simulink model "testboardinternalADC"  (R2018b)
settings: Solver=FixedStepDiscrete  StartTime=0.0  StopTime=Inf  RelTol=1e-3  EnableMultiTasking=on
undefined symbols (not defined in the file or in its folder): Down, GPTRIP1SEL, GPTRIP2SEL, TZ1, TZ2, Up
libraries: c2837xDlib x19, c2802xlib x3, c2000lib x1, simulink x1
settings Model: ExtModeTrigDuration=8  Creator=ThinkPad  LastModifiedBy=ThinkPad
settings OptimizationCC: DefaultUnderspecifiedDataType=single  EnhancedBackFolding=on  PassReuseOutputArgsAs=Individual arguments  MaxStackSize=512  OptimizeBlockOrder=speed  DifferentSizesBufferReuse=on  OptimizationCustomize=off
settings DebuggingCC: ParameterTunabilityLossMsg=error
settings HardwareCC: ProdBitPerChar=16  ProdBitPerInt=16  ProdBitPerPointer=32  ProdBitPerSizeT=32  ProdBitPerPtrDiffT=32  ProdLargestAtomicInteger=Integer  ProdLargestAtomicFloat=None  ProdWordSize=16  ProdLongLongMode=on  ProdHWDeviceType=Texas Instruments->C2000  TargetBitPerChar=16  TargetBitPerInt=16  TargetLargestAtomicInteger=Integer  TargetLongLongMode=on  TargetIntDivRoundTo=Zero  TargetEndianess=LittleEndian  TargetWordSize=16  TargetHWDeviceType=Texas Instruments->C2000
settings SFSimCC: MATLABDynamicMemAlloc=off
settings RTWCC: SystemTargetFile=ert.tlc  HardwareBoard=TI Delfino F2837xD  GenCodeOnly=on  TemplateMakefile=ert_default_tmf  GenerateReport=on  CustomInclude=C:\Users\ThinkPad\Desktop\MBDCODE\  CustomSource=F2837xD_Emif.c  Toolchain=Texas Instruments Code Composer Studio (C2000)  IncludeHyperlinkInReport=on  LaunchReport=on  GenerateTraceInfo=on  GenerateTraceReport=on  GenerateTraceReportSl=on  GenerateTraceReportSf=on  GenerateTraceReportEml=on
settings RTWCC: CustomSourceCode=|
  | //
  | // Globals
  | //
  | Uint16  ErrCount = 0;
  | Uint32  TEST_STATUS;
  | int i;
  | 
  | //
  | // Function Prototypes
  | //
  | extern void setup_emif1_pinmux_async_16bit(Uint16);
  | extern void Emif1Initialize(void);
  | //
  | // mem_read_write - This function performs simple read/write word accesses
  | //                  to memory.
  | //
  | char
  | mem_read_write(Uint32 start_addr, Uint32 mem_size)
  | {
  |     unsigned long mem_rds;
  |     unsigned long mem_wds;
  |     long *XMEM_ps;
  |     unsigned int i;
  | 
  |     //
  |     //Write data
  |     //
  |     XMEM_ps = (long *)start_addr;
  | 
  |     //
  |     //Fill memory
  |     //
  |     mem_wds = 0x01234567;
  |     for (i=0; i < mem_size; i++)
  |     {
  |         *XMEM_ps++ = mem_wds;
  |         mem_wds += 0x11111111;
  |     }
  | 
  |     //
  |     //Verify memory
  |     //
  |     mem_wds = 0x01234567;
  |     XMEM_ps = (long *)start_addr;
  |     for (i=0; i < mem_size; i++)
  |     {
  |         mem_rds = *XMEM_ps;
  |         if( mem_rds != mem_wds)
  |         {
  |             return(1);
  |         }
  |         XMEM_ps++;
  |         mem_wds += 0x11111111;
  |     }
  |     return(0);
  | }
  | 
  | //
  | //  mem_data_walk - This function performs a walking 0 & 1 on data lines for
  | //                  SRAM RD & WR
  | //
  | char
  | mem_data_walk(Uint32 start_addr, Uint32 mem_size)
  | {
  |     unsigned long sram_rd;
  |     unsigned long sram_wd;
  |     unsigned long i;
  |     int k;
  |     int m;
  |     unsigned long  *XM_p;
  |     unsigned long  *XMEM_p;
  | 
  |     XM_p = (unsigned long *)start_addr;
  | 
  |     for (i=0; i < mem_size; i=i+64)
  |     {
  |         for (m=0; m < 2; m++)
  |         {
  |             //
  |             //Write loop
  |             //
  |             XMEM_p = XM_p;
  |             sram_wd = 0x01;
  |             for (k=0; k < 32; k++)
  |             {
  |                 if(m==0)
  |                 {
  |                     *XMEM_p++ =  sram_wd;
  |                 }
  |                 else
  |                 {
  |                     *XMEM_p++ = ~sram_wd;
  |                 }
  |                 sram_wd   = sram_wd<<1;
  |             }
  | 
  |             //
  |             //Read loop
  |             //
  |             XMEM_p = XM_p;
  |             sram_wd = 0x01;
  |             for (k=0; k < 32; k++)
  |             {
  |                 sram_rd = *XMEM_p;
  |                 if(m==1)
  |                 {
  |                     sram_rd = ~sram_rd;
  |                 }
  |                 if(sram_rd != sram_wd)
  |                 {
  |                     return(1);
  |                 }
  |                 XMEM_p++;
  |                 sram_wd=sram_wd<<1;
  |             }
  |         }
  |         XM_p = XMEM_p;
  |     }
  |     return(0);
  | }
  | 
  | //
  | // mem_addr_walk - This function performs a toggle on each address bit.
  | //
  | char
  | mem_addr_walk(Uint32 start_addr, Uint32 addr_size)
  | {
  |     unsigned long sram_rd;
  |     unsigned long sram_wd;
  |     unsigned int k;
  |     unsigned long xshift;
  |     unsigned long  *XM_p;
  |     unsigned long  *XMEM_p;
  | 
  |     XM_p = (unsigned long *)start_addr;
  | 
  |     //
  |     //Write loop
  |     //
  |     xshift = 0x00000001;
  |     sram_wd = 0x00;
  |     for (k=0; k < addr_size; k++)
  |     {
  |         XMEM_p = (unsigned long *)(start_addr + xshift);
  |         *XMEM_p = sram_wd++;
  |         xshift = xshift<<1;
  |     }
  | 
  |     //
  |     //Read loop
  |     //
  |     XMEM_p = XM_p;
  |     xshift = 0x00000001;
  |     sram_wd = 0x00;
  |     for (k=0; k < addr_size; k++)
  |     {
  |         XMEM_p = (unsigned long *)(start_addr + xshift);
  |         sram_rd = *XMEM_p;
  |        if(sram_rd != sram_wd)
  |        {
  |            return(1);
  |        }
  | 
  |        xshift = xshift<<1;
  |        sram_wd++;
  |     }
  |     return(0);
  | }
  | 
  | //
  | // mem_data_size - This function performs different data type
  | //                (HALFWORD/WORD) access.
  | //
  | char
  | mem_data_size(Uint32 start_addr, Uint32 size_to_check)
  | {
  |     unsigned short mem_rds;
  |     unsigned long  mem_rdl;
  |     unsigned short mem_wds;
  |     unsigned long  mem_wdl;
  |     int i;
  | 
  |     short *XMEM_ps;
  |     long  *XMEM_pl;
  | 
  |     //
  |     //Write data short
  |     //
  |     XMEM_ps = (short *)start_addr;
  |     mem_wds = 0x0605;
  | 
  |     for (i=0; i < 2; i++)
  |     {
  |         *XMEM_ps++ = mem_wds;
  |         mem_wds += 0x0202;
  |     }
  | 
  |     //
  |     //Write data long
  |     //
  |     XMEM_pl = (long *)XMEM_ps;
  |     mem_wdl = 0x0C0B0A09;
  |     for (i=0; i < 2; i++)
  |     {
  |         *XMEM_pl++ = mem_wdl;
  |         mem_wdl += 0x04040404;
  |     }
  | 
  |     //
  |     //Read data short
  |     //
  |     XMEM_ps = (short *)start_addr;
  |     mem_wds = 0x0605;
  |     for (i=0; i < 6; i++)
  |     {
  |         mem_rds = *XMEM_ps;
  |         if( mem_rds != mem_wds)
  |         {
  |             return(1);
  |         }
  |         XMEM_ps++;
  |         mem_wds += 0x0202;
  |     }
  | 
  |     //
  |     //Read data long
  |     //
  |     XMEM_pl = (long *)start_addr;
  |     mem_wdl = 0x08070605;
  |     for (i=0; i < 3; i++)
  |     {
  |         mem_rdl = *XMEM_pl;
  |         if(mem_rdl != mem_wdl)
  |         {
  |             return(1);
  |         }
  |         XMEM_pl++;
  |         mem_wdl += 0x04040404;
  |     }
  |     return(0);
  | }
settings RTWCC: CustomHeaderCode=|
  | #include "F28x_Project.h"
  | 
  | #define TEST_PASS            0xABCDABCD
  | #define TEST_FAIL            0xDEADDEAD
  | #define ASRAM_CS3_START_ADDR 0x100000
  | #define ASRAM_CS3_SIZE       0x8000
  | //#define EMIF1                0
  | //#define EMIF2                1
  | #define MEM_D_WIDTH          1            // 16Bit Memory Interface
  | #define TURN_AROUND_TIME     0            // Turn Around time of 2 Emif Clock
  | #define RD_SETUP_TIME        0            // Read Setup time of 1 Emif Clock
  | #define RD_STROBE_TIME       3            // Read Strobe time of 4 Emif Clock
  | #define RD_HOLD_TIME         0            // Read Hold time of 1 Emif Clock
  | #define WR_SETUP_TIME        0            // Write Hold time of 1 Emif Clock
  | #define WR_STROBE_TIME       0            // Write Setup time of 1 Emif Clock
  | #define WR_HOLD_TIME         0            // Write Hold time of 1 Emif Clock
  | #define EXTEND_WAIT          0            // Disable Extended Wait
  | #define STROBE_SEL           0            // Disable Strobe Mode.
  | #define WAIT_POLAR_INV       0
  | #define WAIT_COUNT           0
settings RTWCC: CustomInitializer=|
  | char ErrCount_local;
  |   TEST_STATUS = TEST_FAIL;
  | 
  |   Emif1Initialize();
  |   EALLOW;
  |   CpuSysRegs.PCLKCR1.bit.EMIF1 = 1;
  |   CpuSysRegs.PCLKCR1.bit.EMIF2 = 0;
  |   EDIS;
  |   EALLOW;
  |   ClkCfgRegs.PERCLKDIVSEL.bit.EMIF1CLKDIV = 0x1;
  |   EDIS;
  | 
  |  EALLOW;
  |   ClkCfgRegs.PERCLKDIVSEL.bit.EMIF1CLKDIV = 0x0;
  |   EDIS;
  | 
  |   EALLOW;
  | //
  | // Grab EMIF1 For CPU1
  | //
  |   Emif1ConfigRegs.EMIF1MSEL.all = 0x93A5CE71;
  |   if(Emif1ConfigRegs.EMIF1MSEL.all != 0x1)
  |   {
  |       ErrCount++;
  |   }
  | 
  | //
  | //Disable Access Protection (CPU_FETCH/CPU_WR/DMA_WR)
  | //
  |   Emif1ConfigRegs.EMIF1ACCPROT0.all = 0x0;
  |   if(Emif1ConfigRegs.EMIF1ACCPROT0.all != 0x0)
  |   {
  |       ErrCount++;
  |   }
  | 
  | //
  | // Commit the configuration related to protection. Till this bit remains set
  | // content of EMIF1ACCPROT0 register can't be changed.
  | //
  |   Emif1ConfigRegs.EMIF1COMMIT.all = 0x1;
  |   if(Emif1ConfigRegs.EMIF1COMMIT.all != 0x1)
  |   {
  |      ErrCount++;
  |   }
  | 
  | //
  | // Lock the configuration so that EMIF1COMMIT register can't be
  | // changed any more.
  | //
  |   Emif1ConfigRegs.EMIF1LOCK.all = 0x1;
  |   if(Emif1ConfigRegs.EMIF1LOCK.all != 1)
  |   {
  |       ErrCount++;
  |   }
  | 
  |   EDIS;
  | 
  | 
  | 
  |   EALLOW;
  |   Emif1Regs.RCSR.bit.MODULE_ID = 0x000F;
  |   Emif1Regs.RCSR.bit.FR =1;
  |   EDIS;
  |   EALLOW;
  |   Emif1Regs.ASYNC_WCCR.bit.WP0 = 1;
  |   Emif1Regs.ASYNC_WCCR.bit.MAX_EXT_WAIT = 80;
  |   EDIS;
  |   EALLOW;
  |   Emif1Regs.INT_MSK_SET.bit.AT_MASK_SET = 1;
  |   EDIS;
  | 
  | 
  |     Uint16 i;
  |     for (i=28; i<=37;i++)
  |     {
  |         GPIO_SetupPinMux(i,0,2);
  |     }
  |     for (i=69; i<=83;i++)
  |     {
  |         GPIO_SetupPinMux(i,0,2);
  |     }
  | 
  |     //setup async mode and enable pull-ups for Data pins
  |     for (i=69; i<=83;i++)
  |     {
  |         GPIO_SetupPinOptions(i,0,0x31); // GPIO_ASYNC||GPIO_PULLUP
  |     }
  | 
  | //Configure GPIO pins for EMIF1
  | //
  | //Configure the access timing for CS2 space
  | Emif1Regs.ASYNC_CS3_CR.all =  (EMIF_ASYNC_ASIZE_16    | // 16Bit Memory Interface
  |                              EMIF_ASYNC_TA_4    | // Turn Around time of 2 Emif Clock
  |                              EMIF_ASYNC_RHOLD_4   | // Read Hold time of 1 Emif Clock
  |                              EMIF_ASYNC_RSTROBE_13   | // Read Strobe time of 4 Emif Clock
  |                              EMIF_ASYNC_RSETUP_2  | // Read Setup time of 1 Emif Clock
  |                              EMIF_ASYNC_WHOLD_2   | // Write Hold time of 1 Emif Clock
  |                              EMIF_ASYNC_WSTROBE_7   | // Write Strobe time of 1 Emif Clock
  |                              EMIF_ASYNC_WSETUP_3 | // Write Setup time of 1 Emif Clock
  |                              EMIF_ASYNC_EW_ENABLE  | // Extended Wait Disable.
  |                              EMIF_ASYNC_SS_DISABLE    // Strobe Select Mode Disable.
  |                             );
  | 
  |   ErrCount_local = mem_read_write(ASRAM_CS3_START_ADDR, ASRAM_CS3_SIZE);
  |   ErrCount = ErrCount + ErrCount_local;
  | 
  | //
  | //Address walk checks (Tested for Memory with address width of 16bit)
  | //
  |   ErrCount_local = mem_addr_walk(ASRAM_CS3_START_ADDR, 16);
  |   ErrCount = ErrCount + ErrCount_local;
  | 
  | //
  | //Data walk checks
  | //
  |   ErrCount_local = mem_data_walk(ASRAM_CS3_START_ADDR, ASRAM_CS3_SIZE);
  |   ErrCount = ErrCount + ErrCount_local;
  | 
  | //
  | //Data size checks
  | //
  |   ErrCount_local = mem_data_size(ASRAM_CS3_START_ADDR, 4);
  |   ErrCount = ErrCount + ErrCount_local;
  | 
  |   if (ErrCount == 0x0)
  |   {
  |       TEST_STATUS = TEST_PASS;
  |   }
settings CodeAppCC: ForceParamTrailComments=on  IgnoreCustomStorageClasses=off  OperatorAnnotations=on  SimulinkDataObjDesc=on  SFDataObjDesc=on  InsertBlockDesc=on
settings ERTTargetCC: CodeReplacementLibrary=TI C28x

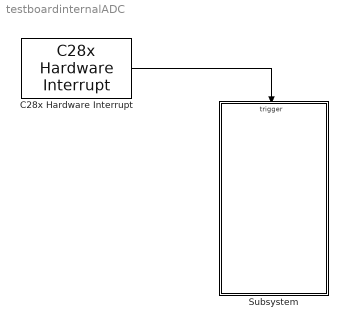
== system testboardinternalADC ==
  C28x Hardware Interrupt : c2000lib/Scheduling/C28x Hardware Interrupt  irqnumbers=[3 3]  pienumbers=[1 2]  irqpriorities=[30 26]  irqpreempts=[0 0]  showinput=off  dspchiptype=C280X
      settings: SourceProductName=Embedded Coder Support Package for Texas Instruments C2000 Processors  SourceProductBaseCode=TIC2000
  Subsystem : Subsystem
  wires:
  C28x Hardware Interrupt/1 -> Subsystem/Trigger

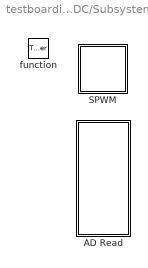
== system testboardinternalADC/Subsystem ==
  function : TriggerPort  TriggerType=function-call  VariantControl=(inherit)  SampleTime=1e-5
  AD Read : Subsystem
  SPWM : Subsystem

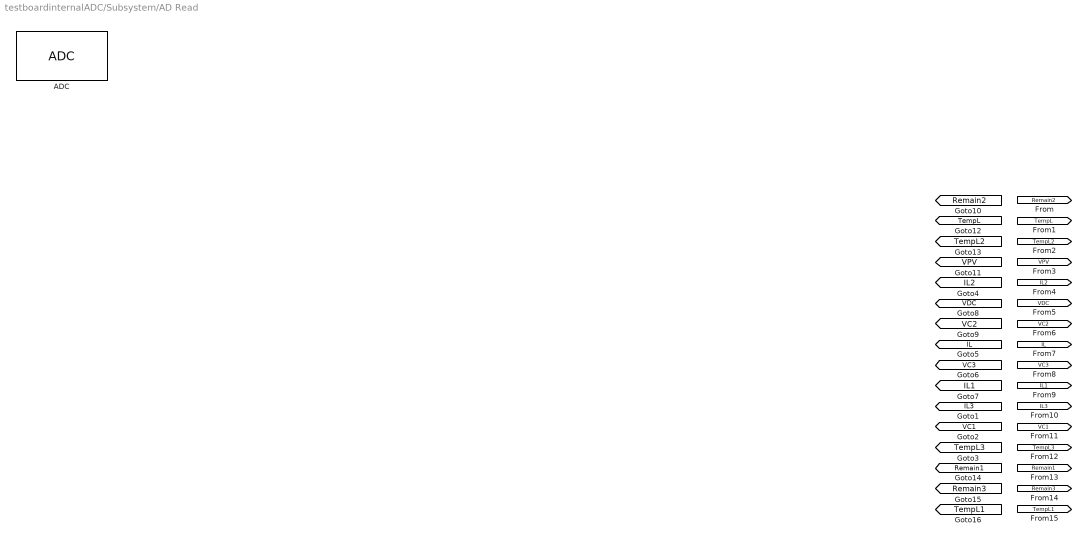
== system testboardinternalADC/Subsystem/AD Read ==
  ADC : c2802xlib/ADC  ADCModule=A  samplingMode=Single sample mode  ADCResolution=12-bit (Single-ended input)  useSOC1=SOC0  useSOC2=SOC0_SOC1  SOCAcquisitionWindow=15  SOCTriggerSource=Software  SOCInterruptTrigger=ADCINT1  Ts=0.001  dType=uint16  postInterrupt=off  interruptSel=ADCINT1  ADCINTContinuous=on  endma=off  chdma=1  blkParamProc=C2000_Type4  conv1=ADCINA0  conv2=ADCINA0 and ADCINB0  conv1_Type4=ADCIN0  conv2_Type4=ADCIN0 and ADCIN1
      settings: SourceProductName=Embedded Coder Support Package for Texas Instruments C2000 Processors
  tag scope: IL1=global, IL2=global, IL3=global, IL=global, Remain1=global, Remain2=global, Remain3=global, TempL1=global, TempL2=global, TempL3=global, TempL=global, VC1=global, VC2=global, VC3=global, VDC=global, VPV=global
  wires:
  ? -> [TempL1]
  ? -> [Remain3]
  ? -> [Remain1]
  ? -> [TempL3]
  ? -> [VC1]
  ? -> [IL1]
  ? -> [VC3]
  ? -> [VC2]
  ? -> [VDC]
  ? -> [TempL2]
  ? -> [IL]
  ? -> [TempL]
  ? -> [VPV]
  ? -> [Remain2]
  ? -> [IL2]
  ? -> [IL3]

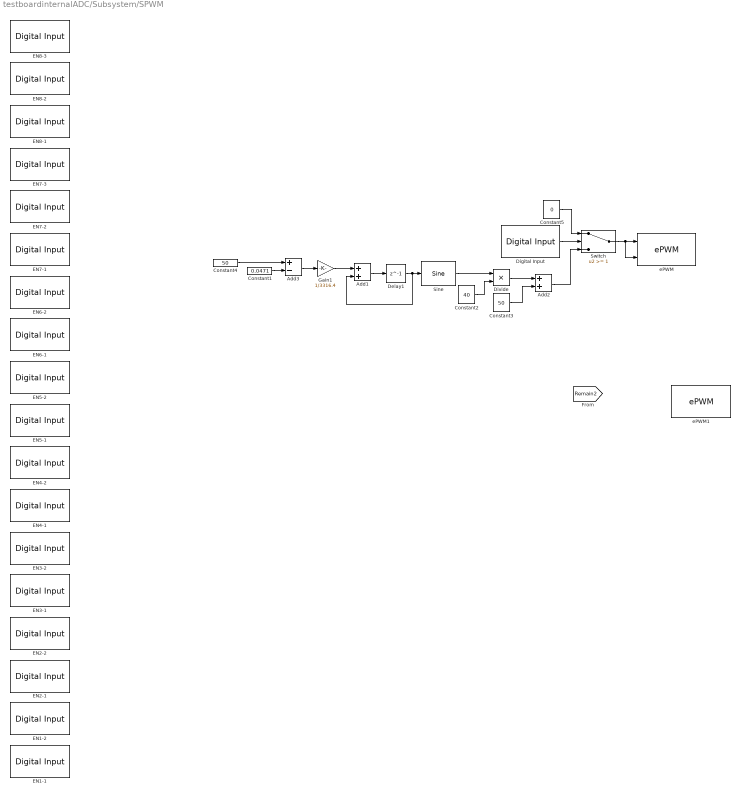
== system testboardinternalADC/Subsystem/SPWM ==
  Add1 : Sum
  Add2 : Sum
  Add3 : Sum  Inputs=+-
  Constant1 : Constant  Value=0.0471  VectorParams1D=off
  Constant2 : Constant  Value=40  VectorParams1D=off
  Constant3 : Constant  Value=50  VectorParams1D=off
  Constant4 : Constant  Value=50  VectorParams1D=off
  Constant5 : Constant  Value=0  VectorParams1D=off
  Delay1 : Delay  DelayLength=1
  Digital Input : c2837xDlib/Digital Input  GPIO_Number=GPIO96~GPIO103  GPIO_Bit0=off  GPIO_Bit1=off  GPIO_Bit2=off  GPIO_Bit3=on  GPIO_Bit4=off  GPIO_Bit5=off  GPIO_Bit6=off  GPIO_Bit7=off  sampleTime=-1  dataType=auto  GPIO_Bit0_Qualification=Sync to SYSCLKOUT  GPIO_Bit1_Qualification=Sync to SYSCLKOUT  GPIO_Bit2_Qualification=Sync to SYSCLKOUT  GPIO_Bit3_Qualification=Sync to SYSCLKOUT  GPIO_Bit4_Qualification=Sync to SYSCLKOUT  GPIO_Bit5_Qualification=Sync to SYSCLKOUT  GPIO_Bit6_Qualification=Sync to SYSCLKOUT  GPIO_Bit7_Qualification=Sync to SYSCLKOUT  Qualification_Period=-1
      settings: SourceProductName=Embedded Coder Support Package for Texas Instruments C2000 Processors  SourceProductBaseCode=TIC2000
  Divide : Product  Inputs=**
  EN1-1 : c2837xDlib/Digital Input  GPIO_Number=GPIO88~GPIO95  GPIO_Bit0=off  GPIO_Bit1=off  GPIO_Bit2=on  GPIO_Bit3=off  GPIO_Bit4=off  GPIO_Bit5=off  GPIO_Bit6=off  GPIO_Bit7=off  sampleTime=0.1  dataType=auto  GPIO_Bit0_Qualification=Sync to SYSCLKOUT  GPIO_Bit1_Qualification=Sync to SYSCLKOUT  GPIO_Bit2_Qualification=Sync to SYSCLKOUT  GPIO_Bit3_Qualification=Sync to SYSCLKOUT  GPIO_Bit4_Qualification=Sync to SYSCLKOUT  GPIO_Bit5_Qualification=Sync to SYSCLKOUT  GPIO_Bit6_Qualification=Sync to SYSCLKOUT  GPIO_Bit7_Qualification=Sync to SYSCLKOUT  Qualification_Period=-1
      settings: SourceProductName=Embedded Coder Support Package for Texas Instruments C2000 Processors  SourceProductBaseCode=TIC2000
  EN1-2 : c2837xDlib/Digital Input  GPIO_Number=GPIO88~GPIO95  GPIO_Bit0=off  GPIO_Bit1=on  GPIO_Bit2=off  GPIO_Bit3=off  GPIO_Bit4=off  GPIO_Bit5=off  GPIO_Bit6=off  GPIO_Bit7=off  sampleTime=0.1  dataType=auto  GPIO_Bit0_Qualification=Sync to SYSCLKOUT  GPIO_Bit1_Qualification=Sync to SYSCLKOUT  GPIO_Bit2_Qualification=Sync to SYSCLKOUT  GPIO_Bit3_Qualification=Sync to SYSCLKOUT  GPIO_Bit4_Qualification=Sync to SYSCLKOUT  GPIO_Bit5_Qualification=Sync to SYSCLKOUT  GPIO_Bit6_Qualification=Sync to SYSCLKOUT  GPIO_Bit7_Qualification=Sync to SYSCLKOUT  Qualification_Period=-1
      settings: SourceProductName=Embedded Coder Support Package for Texas Instruments C2000 Processors  SourceProductBaseCode=TIC2000
  EN2-1 : c2837xDlib/Digital Input  GPIO_Number=GPIO88~GPIO95  GPIO_Bit0=on  GPIO_Bit1=off  GPIO_Bit2=off  GPIO_Bit3=off  GPIO_Bit4=off  GPIO_Bit5=off  GPIO_Bit6=off  GPIO_Bit7=off  sampleTime=0.1  dataType=auto  GPIO_Bit0_Qualification=Sync to SYSCLKOUT  GPIO_Bit1_Qualification=Sync to SYSCLKOUT  GPIO_Bit2_Qualification=Sync to SYSCLKOUT  GPIO_Bit3_Qualification=Sync to SYSCLKOUT  GPIO_Bit4_Qualification=Sync to SYSCLKOUT  GPIO_Bit5_Qualification=Sync to SYSCLKOUT  GPIO_Bit6_Qualification=Sync to SYSCLKOUT  GPIO_Bit7_Qualification=Sync to SYSCLKOUT  Qualification_Period=-1
      settings: SourceProductName=Embedded Coder Support Package for Texas Instruments C2000 Processors  SourceProductBaseCode=TIC2000
  EN2-2 : c2837xDlib/Digital Input  GPIO_Number=GPIO80~GPIO87  GPIO_Bit0=off  GPIO_Bit1=off  GPIO_Bit2=off  GPIO_Bit3=off  GPIO_Bit4=off  GPIO_Bit5=off  GPIO_Bit6=off  GPIO_Bit7=on  sampleTime=0.1  dataType=auto  GPIO_Bit0_Qualification=Sync to SYSCLKOUT  GPIO_Bit1_Qualification=Sync to SYSCLKOUT  GPIO_Bit2_Qualification=Sync to SYSCLKOUT  GPIO_Bit3_Qualification=Sync to SYSCLKOUT  GPIO_Bit4_Qualification=Sync to SYSCLKOUT  GPIO_Bit5_Qualification=Sync to SYSCLKOUT  GPIO_Bit6_Qualification=Sync to SYSCLKOUT  GPIO_Bit7_Qualification=Sync to SYSCLKOUT  Qualification_Period=-1
      settings: SourceProductName=Embedded Coder Support Package for Texas Instruments C2000 Processors  SourceProductBaseCode=TIC2000
  EN3-1 : c2837xDlib/Digital Input  GPIO_Number=GPIO80~GPIO87  GPIO_Bit0=off  GPIO_Bit1=off  GPIO_Bit2=off  GPIO_Bit3=off  GPIO_Bit4=off  GPIO_Bit5=off  GPIO_Bit6=on  GPIO_Bit7=off  sampleTime=0.1  dataType=auto  GPIO_Bit0_Qualification=Sync to SYSCLKOUT  GPIO_Bit1_Qualification=Sync to SYSCLKOUT  GPIO_Bit2_Qualification=Sync to SYSCLKOUT  GPIO_Bit3_Qualification=Sync to SYSCLKOUT  GPIO_Bit4_Qualification=Sync to SYSCLKOUT  GPIO_Bit5_Qualification=Sync to SYSCLKOUT  GPIO_Bit6_Qualification=Sync to SYSCLKOUT  GPIO_Bit7_Qualification=Sync to SYSCLKOUT  Qualification_Period=-1
      settings: SourceProductName=Embedded Coder Support Package for Texas Instruments C2000 Processors  SourceProductBaseCode=TIC2000
  EN3-2 : c2837xDlib/Digital Input  GPIO_Number=GPIO48~GPIO55  GPIO_Bit0=off  GPIO_Bit1=off  GPIO_Bit2=off  GPIO_Bit3=off  GPIO_Bit4=on  GPIO_Bit5=off  GPIO_Bit6=off  GPIO_Bit7=off  sampleTime=0.1  dataType=auto  GPIO_Bit0_Qualification=Sync to SYSCLKOUT  GPIO_Bit1_Qualification=Sync to SYSCLKOUT  GPIO_Bit2_Qualification=Sync to SYSCLKOUT  GPIO_Bit3_Qualification=Sync to SYSCLKOUT  GPIO_Bit4_Qualification=Sync to SYSCLKOUT  GPIO_Bit5_Qualification=Sync to SYSCLKOUT  GPIO_Bit6_Qualification=Sync to SYSCLKOUT  GPIO_Bit7_Qualification=Sync to SYSCLKOUT  Qualification_Period=-1
      settings: SourceProductName=Embedded Coder Support Package for Texas Instruments C2000 Processors  SourceProductBaseCode=TIC2000
  EN4-1 : c2837xDlib/Digital Input  GPIO_Number=GPIO48~GPIO55  GPIO_Bit0=off  GPIO_Bit1=off  GPIO_Bit2=off  GPIO_Bit3=on  GPIO_Bit4=off  GPIO_Bit5=off  GPIO_Bit6=off  GPIO_Bit7=off  sampleTime=0.1  dataType=auto  GPIO_Bit0_Qualification=Sync to SYSCLKOUT  GPIO_Bit1_Qualification=Sync to SYSCLKOUT  GPIO_Bit2_Qualification=Sync to SYSCLKOUT  GPIO_Bit3_Qualification=Sync to SYSCLKOUT  GPIO_Bit4_Qualification=Sync to SYSCLKOUT  GPIO_Bit5_Qualification=Sync to SYSCLKOUT  GPIO_Bit6_Qualification=Sync to SYSCLKOUT  GPIO_Bit7_Qualification=Sync to SYSCLKOUT  Qualification_Period=-1
      settings: SourceProductName=Embedded Coder Support Package for Texas Instruments C2000 Processors  SourceProductBaseCode=TIC2000
  EN4-2 : c2837xDlib/Digital Input  GPIO_Number=GPIO48~GPIO55  GPIO_Bit0=off  GPIO_Bit1=off  GPIO_Bit2=on  GPIO_Bit3=off  GPIO_Bit4=off  GPIO_Bit5=off  GPIO_Bit6=off  GPIO_Bit7=off  sampleTime=0.1  dataType=auto  GPIO_Bit0_Qualification=Sync to SYSCLKOUT  GPIO_Bit1_Qualification=Sync to SYSCLKOUT  GPIO_Bit2_Qualification=Sync to SYSCLKOUT  GPIO_Bit3_Qualification=Sync to SYSCLKOUT  GPIO_Bit4_Qualification=Sync to SYSCLKOUT  GPIO_Bit5_Qualification=Sync to SYSCLKOUT  GPIO_Bit6_Qualification=Sync to SYSCLKOUT  GPIO_Bit7_Qualification=Sync to SYSCLKOUT  Qualification_Period=-1
      settings: SourceProductName=Embedded Coder Support Package for Texas Instruments C2000 Processors  SourceProductBaseCode=TIC2000
  EN5-1 : c2837xDlib/Digital Input  GPIO_Number=GPIO48~GPIO55  GPIO_Bit0=off  GPIO_Bit1=on  GPIO_Bit2=off  GPIO_Bit3=off  GPIO_Bit4=off  GPIO_Bit5=off  GPIO_Bit6=off  GPIO_Bit7=off  sampleTime=0.1  dataType=auto  GPIO_Bit0_Qualification=Sync to SYSCLKOUT  GPIO_Bit1_Qualification=Sync to SYSCLKOUT  GPIO_Bit2_Qualification=Sync to SYSCLKOUT  GPIO_Bit3_Qualification=Sync to SYSCLKOUT  GPIO_Bit4_Qualification=Sync to SYSCLKOUT  GPIO_Bit5_Qualification=Sync to SYSCLKOUT  GPIO_Bit6_Qualification=Sync to SYSCLKOUT  GPIO_Bit7_Qualification=Sync to SYSCLKOUT  Qualification_Period=-1
      settings: SourceProductName=Embedded Coder Support Package for Texas Instruments C2000 Processors  SourceProductBaseCode=TIC2000
  EN5-2 : c2837xDlib/Digital Input  GPIO_Number=GPIO48~GPIO55  GPIO_Bit0=on  GPIO_Bit1=off  GPIO_Bit2=off  GPIO_Bit3=off  GPIO_Bit4=off  GPIO_Bit5=off  GPIO_Bit6=off  GPIO_Bit7=off  sampleTime=0.1  dataType=auto  GPIO_Bit0_Qualification=Sync to SYSCLKOUT  GPIO_Bit1_Qualification=Sync to SYSCLKOUT  GPIO_Bit2_Qualification=Sync to SYSCLKOUT  GPIO_Bit3_Qualification=Sync to SYSCLKOUT  GPIO_Bit4_Qualification=Sync to SYSCLKOUT  GPIO_Bit5_Qualification=Sync to SYSCLKOUT  GPIO_Bit6_Qualification=Sync to SYSCLKOUT  GPIO_Bit7_Qualification=Sync to SYSCLKOUT  Qualification_Period=-1
      settings: SourceProductName=Embedded Coder Support Package for Texas Instruments C2000 Processors  SourceProductBaseCode=TIC2000
  EN6-1 : c2837xDlib/Digital Input  GPIO_Number=GPIO40~GPIO47  GPIO_Bit0=off  GPIO_Bit1=off  GPIO_Bit2=off  GPIO_Bit3=off  GPIO_Bit4=off  GPIO_Bit5=off  GPIO_Bit6=off  GPIO_Bit7=on  sampleTime=0.1  dataType=auto  GPIO_Bit0_Qualification=Sync to SYSCLKOUT  GPIO_Bit1_Qualification=Sync to SYSCLKOUT  GPIO_Bit2_Qualification=Sync to SYSCLKOUT  GPIO_Bit3_Qualification=Sync to SYSCLKOUT  GPIO_Bit4_Qualification=Sync to SYSCLKOUT  GPIO_Bit5_Qualification=Sync to SYSCLKOUT  GPIO_Bit6_Qualification=Sync to SYSCLKOUT  GPIO_Bit7_Qualification=Sync to SYSCLKOUT  Qualification_Period=-1
      settings: SourceProductName=Embedded Coder Support Package for Texas Instruments C2000 Processors  SourceProductBaseCode=TIC2000
  EN6-2 : c2837xDlib/Digital Input  GPIO_Number=GPIO40~GPIO47  GPIO_Bit0=off  GPIO_Bit1=off  GPIO_Bit2=off  GPIO_Bit3=off  GPIO_Bit4=off  GPIO_Bit5=off  GPIO_Bit6=on  GPIO_Bit7=off  sampleTime=0.1  dataType=auto  GPIO_Bit0_Qualification=Sync to SYSCLKOUT  GPIO_Bit1_Qualification=Sync to SYSCLKOUT  GPIO_Bit2_Qualification=Sync to SYSCLKOUT  GPIO_Bit3_Qualification=Sync to SYSCLKOUT  GPIO_Bit4_Qualification=Sync to SYSCLKOUT  GPIO_Bit5_Qualification=Sync to SYSCLKOUT  GPIO_Bit6_Qualification=Sync to SYSCLKOUT  GPIO_Bit7_Qualification=Sync to SYSCLKOUT  Qualification_Period=-1
      settings: SourceProductName=Embedded Coder Support Package for Texas Instruments C2000 Processors  SourceProductBaseCode=TIC2000
  EN7-1 : c2837xDlib/Digital Input  GPIO_Number=GPIO40~GPIO47  GPIO_Bit0=off  GPIO_Bit1=off  GPIO_Bit2=off  GPIO_Bit3=off  GPIO_Bit4=off  GPIO_Bit5=on  GPIO_Bit6=off  GPIO_Bit7=off  sampleTime=0.1  dataType=auto  GPIO_Bit0_Qualification=Sync to SYSCLKOUT  GPIO_Bit1_Qualification=Sync to SYSCLKOUT  GPIO_Bit2_Qualification=Sync to SYSCLKOUT  GPIO_Bit3_Qualification=Sync to SYSCLKOUT  GPIO_Bit4_Qualification=Sync to SYSCLKOUT  GPIO_Bit5_Qualification=Sync to SYSCLKOUT  GPIO_Bit6_Qualification=Sync to SYSCLKOUT  GPIO_Bit7_Qualification=Sync to SYSCLKOUT  Qualification_Period=-1
      settings: SourceProductName=Embedded Coder Support Package for Texas Instruments C2000 Processors  SourceProductBaseCode=TIC2000
  EN7-2 : c2837xDlib/Digital Input  GPIO_Number=GPIO40~GPIO47  GPIO_Bit0=off  GPIO_Bit1=off  GPIO_Bit2=off  GPIO_Bit3=off  GPIO_Bit4=on  GPIO_Bit5=off  GPIO_Bit6=off  GPIO_Bit7=off  sampleTime=0.1  dataType=auto  GPIO_Bit0_Qualification=Sync to SYSCLKOUT  GPIO_Bit1_Qualification=Sync to SYSCLKOUT  GPIO_Bit2_Qualification=Sync to SYSCLKOUT  GPIO_Bit3_Qualification=Sync to SYSCLKOUT  GPIO_Bit4_Qualification=Sync to SYSCLKOUT  GPIO_Bit5_Qualification=Sync to SYSCLKOUT  GPIO_Bit6_Qualification=Sync to SYSCLKOUT  GPIO_Bit7_Qualification=Sync to SYSCLKOUT  Qualification_Period=-1
      settings: SourceProductName=Embedded Coder Support Package for Texas Instruments C2000 Processors  SourceProductBaseCode=TIC2000
  EN7-3 : c2837xDlib/Digital Input  GPIO_Number=GPIO40~GPIO47  GPIO_Bit0=off  GPIO_Bit1=on  GPIO_Bit2=off  GPIO_Bit3=off  GPIO_Bit4=off  GPIO_Bit5=off  GPIO_Bit6=off  GPIO_Bit7=off  sampleTime=0.1  dataType=auto  GPIO_Bit0_Qualification=Sync to SYSCLKOUT  GPIO_Bit1_Qualification=Sync to SYSCLKOUT  GPIO_Bit2_Qualification=Sync to SYSCLKOUT  GPIO_Bit3_Qualification=Sync to SYSCLKOUT  GPIO_Bit4_Qualification=Sync to SYSCLKOUT  GPIO_Bit5_Qualification=Sync to SYSCLKOUT  GPIO_Bit6_Qualification=Sync to SYSCLKOUT  GPIO_Bit7_Qualification=Sync to SYSCLKOUT  Qualification_Period=-1
      settings: SourceProductName=Embedded Coder Support Package for Texas Instruments C2000 Processors  SourceProductBaseCode=TIC2000
  EN8-1 : c2837xDlib/Digital Input  GPIO_Number=GPIO40~GPIO47  GPIO_Bit0=on  GPIO_Bit1=off  GPIO_Bit2=off  GPIO_Bit3=off  GPIO_Bit4=off  GPIO_Bit5=off  GPIO_Bit6=off  GPIO_Bit7=off  sampleTime=0.1  dataType=auto  GPIO_Bit0_Qualification=Sync to SYSCLKOUT  GPIO_Bit1_Qualification=Sync to SYSCLKOUT  GPIO_Bit2_Qualification=Sync to SYSCLKOUT  GPIO_Bit3_Qualification=Sync to SYSCLKOUT  GPIO_Bit4_Qualification=Sync to SYSCLKOUT  GPIO_Bit5_Qualification=Sync to SYSCLKOUT  GPIO_Bit6_Qualification=Sync to SYSCLKOUT  GPIO_Bit7_Qualification=Sync to SYSCLKOUT  Qualification_Period=-1
      settings: SourceProductName=Embedded Coder Support Package for Texas Instruments C2000 Processors  SourceProductBaseCode=TIC2000
  EN8-2 : c2837xDlib/Digital Input  GPIO_Number=GPIO32~GPIO39  GPIO_Bit0=off  GPIO_Bit1=off  GPIO_Bit2=off  GPIO_Bit3=off  GPIO_Bit4=off  GPIO_Bit5=off  GPIO_Bit6=off  GPIO_Bit7=on  sampleTime=0.1  dataType=auto  GPIO_Bit0_Qualification=Sync to SYSCLKOUT  GPIO_Bit1_Qualification=Sync to SYSCLKOUT  GPIO_Bit2_Qualification=Sync to SYSCLKOUT  GPIO_Bit3_Qualification=Sync to SYSCLKOUT  GPIO_Bit4_Qualification=Sync to SYSCLKOUT  GPIO_Bit5_Qualification=Sync to SYSCLKOUT  GPIO_Bit6_Qualification=Sync to SYSCLKOUT  GPIO_Bit7_Qualification=Sync to SYSCLKOUT  Qualification_Period=-1
      settings: SourceProductName=Embedded Coder Support Package for Texas Instruments C2000 Processors  SourceProductBaseCode=TIC2000
  EN8-3 : c2837xDlib/Digital Input  GPIO_Number=GPIO32~GPIO39  GPIO_Bit0=off  GPIO_Bit1=off  GPIO_Bit2=off  GPIO_Bit3=off  GPIO_Bit4=off  GPIO_Bit5=off  GPIO_Bit6=on  GPIO_Bit7=off  sampleTime=0.1  dataType=auto  GPIO_Bit0_Qualification=Sync to SYSCLKOUT  GPIO_Bit1_Qualification=Sync to SYSCLKOUT  GPIO_Bit2_Qualification=Sync to SYSCLKOUT  GPIO_Bit3_Qualification=Sync to SYSCLKOUT  GPIO_Bit4_Qualification=Sync to SYSCLKOUT  GPIO_Bit5_Qualification=Sync to SYSCLKOUT  GPIO_Bit6_Qualification=Sync to SYSCLKOUT  GPIO_Bit7_Qualification=Sync to SYSCLKOUT  Qualification_Period=-1
      settings: SourceProductName=Embedded Coder Support Package for Texas Instruments C2000 Processors  SourceProductBaseCode=TIC2000
  Gain1 : Gain  Gain=1/3316.4
  Sine : simulink/Lookup Tables/Sine  Formula=sin(2*pi*u)  NumDataPoints=(2^8)+1  OutputWordLength=16  InternalRulePriority=Speed
      settings: SourceProductName=Simulink
  Switch : Switch  Threshold=1
  ePWM : c2802xlib/ePWM  useModule=ePWM1  ePWMxLINKTBPRD=Not Linked  periodUnits=Clock cycles  timerSource=Specify via dialog  timerPeriod_clk=15000  timerPeriod_sec=0.0001  tbshadow=Counter equals to zero  countingMode=Up-Down  phaseActiveEnable=Disable  phaseDirection=Count down after sync  phaseActive=0  synchronizationEnable=off  dcaevt1Sync=off  dcbevt1Sync=off  synchronizationOption=Disable  clockPrescale=1  HSclockPrescale=1  enswap=off  ePWMxAStatus=on  ePWMxAactionLogic1=Set  ePWMxAactionLogic2=Clear  ePWMxAactionLogic3=Clear  ePWMxAactionLogic4=Set  ePWMxAactionLogic5=Do nothing  ePWMxAactionLogic6=Do nothing  ePWMxALoadMode=Load on counter equals to zero (CTR=Zero)  ePWMxACSFenable=off  ePWMxACSFvalue=Forcing disable  ePWMxASFreload=Zero  ePWMxBStatus=on  ePWMxBactionLogic1=Set  ePWMxBactionLogic2=Clear  ePWMxBactionLogic3=Do nothing  ePWMxBactionLogic4=Do nothing  ePWMxBactionLogic5=Clear  ePWMxBactionLogic6=Set  ePWMxBLoadMode=Load on counter equals to zero (CTR=Zero)  ePWMxBCSFenable=off  ePWMxBCSFvalue=Forcing disable  ePWMxBSFreload=Zero  ePWNxBOutWay=on  ePWMxLINKCMPA=Not Linked  CMPAUnits=Percentages  CMPASource=Input port  CMPAValue_per=0  CMPAValue_clk=0  enCMPAshadow=Counter equals to zero  ePWMxLINKCMPB=Not Linked  CMPBUnits=Percentages  CMPBSource=Input port  CMPBValue_per=0  CMPBValue_clk=0  enCMPBshadow=Counter equals to zero  ePWMxLINKCMPC=Not Linked  CMPCUnits=Clock cycles  CMPCSource=Specify via dialog  CMPCValue_per=50  CMPCValue_clk=32000  enCMPCshadow=Counter equals to zero  ePWMxLINKCMPD=Not Linked  CMPDUnits=Clock cycles  CMPDSource=Specify via dialog  CMPDValue_per=50  CMPDValue_clk=32000  enCMPDshadow=Counter equals to zero  enableDBePWMxA=on  enableDBePWMxB=on  enhalfcycle=off  DBpolarity=Active high (AH)  DBedgeDelay=Positive  DBSource_ePWMxA=ePWMxA  DBSource_ePWMxB=ePWMxA  DBperiodSource=Specify via dialog  REDperiod=500  FEDperiod=500  adcstartModuleA=off  adcrequestEventA=First event  adcstartEventA=Digital Compare Module A Event 1 start of conversion (DCAEVT1.soc)  adcstartEventA_type2=Digital Compare Module A Event 1 start of conversion (DCAEVT1.soc)  adcstartModuleB=off  adcrequestEventB=First event  adcstartEventB=Counter equals to zero (CTR=Zero)  adcstartEventB_type2=Counter equals to zero (CTR=Zero)  intEn=on  intPrd=First event  intSel=Counter equals to zero (CTR=Zero)  intSel_type2=Counter equals to zero (CTR=Zero)  hrpe=off  enHRPWM=off  HRPWM_LoadMode=Counter equals to period (CTR=PRD)  HRPWM_CTLMode=Duty or Period control mode  HRPWM_EDGMode=Both edge  hrpeb=off  enHRPWMB=off  HRPWM_LoadModeB=Counter equals to zero (CTR=ZERO)  HRPWM_CTLModeB=Duty or Period control mode  HRPWM_EDGModeB=Both edge  enSFO=on  enautoconv=on  chopperEnable=off  chopperFrequency=1  chopperFirstwidth=1  chopperDuty=12.5%  tripZonesource=Specify via dialog  tzselOSHT1=off  tzselOSHT2=off  tzselOSHT3=off  tzselOSHDCAEV1=off  tzselOSHDCBEV1=off  tzselCBC1=off  tzselCBC2=off  tzselCBC3=off  tzselCBCDCAEV2=off  tzselCBCDCBEV2=off  tzselOSHT4=off  tzselOSHT5=off  tzselOSHT6=off  tzselCBC4=off  tzselCBC5=off  tzselCBC6=off  enTzOstIntr=off  enTzCbcIntr=off  enTzDCAEVT1Intr=off  enTzDCAEVT2Intr=off  enTzDCBEVT1Intr=off  enTzDCBEVT2Intr=off  ePWMxAforced=No action  ePWMxBforced=No action  DCAEVT1forced=No action  DCBEVT1forced=No action  DCAEVT2forced=No action  DCBEVT2forced=No action  dcah=Trip Zone 1 input (TZ1)  dcal=Trip Zone 2 input (TZ2)  dcbh=Trip Zone 1 input (TZ1)  dcbl=Trip Zone 2 input (TZ2)  dcah_type2=GPTRIP1SEL/(TZ1)  dcal_type2=GPTRIP2SEL/(TZ2)  dcbh_type2=GPTRIP1SEL/(TZ1)  dcbl_type2=GPTRIP2SEL/(TZ2)  gendcaevt1=Event disabled  gendcaevt2=Event disabled  gendcbevt1=Event disabled  gendcbevt2=Event disabled  dcaevt1src=DCAEVT1 with sync  dcaevt2src=DCAEVT2 with sync  dcbevt1src=DCBEVT1 with sync  dcbevt2src=DCBEVT2 with sync  pulsesel=Counter equals to zero (CTR=Zero)  blankinv=off  blankoffset=0  blankwidth=0  evsrcsel=Filtered version of DCAEVT1 (DCAEVT1FILT)  encape=off  PwmType=C2000_Type4
      settings: SourceProductName=Embedded Coder Support Package for Texas Instruments C2000 Processors
  ePWM1 : c2802xlib/ePWM  useModule=ePWM2  ePWMxLINKTBPRD=Not Linked  periodUnits=Clock cycles  timerSource=Specify via dialog  timerPeriod_clk=15000  timerPeriod_sec=0.0001  tbshadow=Counter equals to zero  countingMode=Up-Down  phaseActiveEnable=Disable  phaseDirection=Count down after sync  phaseActive=0  synchronizationEnable=off  dcaevt1Sync=off  dcbevt1Sync=off  synchronizationOption=Disable  clockPrescale=1  HSclockPrescale=1  enswap=off  ePWMxAStatus=on  ePWMxAactionLogic1=Set  ePWMxAactionLogic2=Clear  ePWMxAactionLogic3=Clear  ePWMxAactionLogic4=Set  ePWMxAactionLogic5=Do nothing  ePWMxAactionLogic6=Do nothing  ePWMxALoadMode=Load on counter equals to zero (CTR=Zero)  ePWMxACSFenable=off  ePWMxACSFvalue=Forcing disable  ePWMxASFreload=Zero  ePWMxBStatus=on  ePWMxBactionLogic1=Set  ePWMxBactionLogic2=Clear  ePWMxBactionLogic3=Do nothing  ePWMxBactionLogic4=Do nothing  ePWMxBactionLogic5=Clear  ePWMxBactionLogic6=Set  ePWMxBLoadMode=Load on counter equals to zero (CTR=Zero)  ePWMxBCSFenable=off  ePWMxBCSFvalue=Forcing disable  ePWMxBSFreload=Zero  ePWNxBOutWay=on  ePWMxLINKCMPA=Not Linked  CMPAUnits=Percentages  CMPASource=Input port  CMPAValue_per=0  CMPAValue_clk=0  enCMPAshadow=Counter equals to zero  ePWMxLINKCMPB=Not Linked  CMPBUnits=Percentages  CMPBSource=Input port  CMPBValue_per=0  CMPBValue_clk=0  enCMPBshadow=Counter equals to zero  ePWMxLINKCMPC=Not Linked  CMPCUnits=Clock cycles  CMPCSource=Specify via dialog  CMPCValue_per=50  CMPCValue_clk=32000  enCMPCshadow=Counter equals to zero  ePWMxLINKCMPD=Not Linked  CMPDUnits=Clock cycles  CMPDSource=Specify via dialog  CMPDValue_per=50  CMPDValue_clk=32000  enCMPDshadow=Counter equals to zero  enableDBePWMxA=on  enableDBePWMxB=on  enhalfcycle=off  DBpolarity=Active high (AH)  DBedgeDelay=Positive  DBSource_ePWMxA=ePWMxA  DBSource_ePWMxB=ePWMxA  DBperiodSource=Specify via dialog  REDperiod=500  FEDperiod=500  adcstartModuleA=off  adcrequestEventA=First event  adcstartEventA=Digital Compare Module A Event 1 start of conversion (DCAEVT1.soc)  adcstartEventA_type2=Digital Compare Module A Event 1 start of conversion (DCAEVT1.soc)  adcstartModuleB=off  adcrequestEventB=First event  adcstartEventB=Counter equals to zero (CTR=Zero)  adcstartEventB_type2=Counter equals to zero (CTR=Zero)  intEn=on  intPrd=First event  intSel=Counter equals to zero (CTR=Zero)  intSel_type2=Counter equals to zero (CTR=Zero)  hrpe=off  enHRPWM=off  HRPWM_LoadMode=Counter equals to period (CTR=PRD)  HRPWM_CTLMode=Duty or Period control mode  HRPWM_EDGMode=Both edge  hrpeb=off  enHRPWMB=off  HRPWM_LoadModeB=Counter equals to zero (CTR=ZERO)  HRPWM_CTLModeB=Duty or Period control mode  HRPWM_EDGModeB=Both edge  enSFO=on  enautoconv=on  chopperEnable=off  chopperFrequency=1  chopperFirstwidth=1  chopperDuty=12.5%  tripZonesource=Specify via dialog  tzselOSHT1=off  tzselOSHT2=off  tzselOSHT3=off  tzselOSHDCAEV1=off  tzselOSHDCBEV1=off  tzselCBC1=off  tzselCBC2=off  tzselCBC3=off  tzselCBCDCAEV2=off  tzselCBCDCBEV2=off  tzselOSHT4=off  tzselOSHT5=off  tzselOSHT6=off  tzselCBC4=off  tzselCBC5=off  tzselCBC6=off  enTzOstIntr=off  enTzCbcIntr=off  enTzDCAEVT1Intr=off  enTzDCAEVT2Intr=off  enTzDCBEVT1Intr=off  enTzDCBEVT2Intr=off  ePWMxAforced=No action  ePWMxBforced=No action  DCAEVT1forced=No action  DCBEVT1forced=No action  DCAEVT2forced=No action  DCBEVT2forced=No action  dcah=Trip Zone 1 input (TZ1)  dcal=Trip Zone 2 input (TZ2)  dcbh=Trip Zone 1 input (TZ1)  dcbl=Trip Zone 2 input (TZ2)  dcah_type2=GPTRIP1SEL/(TZ1)  dcal_type2=GPTRIP2SEL/(TZ2)  dcbh_type2=GPTRIP1SEL/(TZ1)  dcbl_type2=GPTRIP2SEL/(TZ2)  gendcaevt1=Event disabled  gendcaevt2=Event disabled  gendcbevt1=Event disabled  gendcbevt2=Event disabled  dcaevt1src=DCAEVT1 with sync  dcaevt2src=DCAEVT2 with sync  dcbevt1src=DCBEVT1 with sync  dcbevt2src=DCBEVT2 with sync  pulsesel=Counter equals to zero (CTR=Zero)  blankinv=off  blankoffset=0  blankwidth=0  evsrcsel=Filtered version of DCAEVT1 (DCAEVT1FILT)  encape=off  PwmType=C2000_Type4
      settings: SourceProductName=Embedded Coder Support Package for Texas Instruments C2000 Processors
  wires:
  Sine/1 -> Divide/1
  Divide/1 -> Add2/1
  Add3/1 -> Gain1/1
  Constant1/1 -> Add3/2
  Constant3/1 -> Add2/2
  Constant4/1 -> Add3/1
  Delay1/1 -> Sine/1, Add1/2
  Constant2/1 -> Divide/2
  Gain1/1 -> Add1/1
  Add1/1 -> Delay1/1
  Digital Input/1 -> Switch/2
  Constant5/1 -> Switch/1
  Add2/1 -> Switch/3
  Switch/1 -> ePWM/2, ePWM/1
